simulink model "robotsim"  (Simulink 7.4)
settings: Solver=ode45  StartTime=0.0  StopTime=0.05  FixedStep=0.01  MaxStep=0.01  MinStep=0.001  RelTol=1e-3
values from neighbouring files (symbols this model uses):
  robot = wam    [WAMforcecontrol.m]    (also in batchwamobs.m; controltest.m; feedforward.m; inertia2.m = p560)
  uc = M*y+N    [WAMforcecontrol.m]    (also in controltest.m = y+uest; feedforward.m = M*ddqd(i,:)'+Nd; observerest.m = u(1:n); observerest2.m = u(1:n))
  uest = zeros(n,1)    [WAMforcecontrol.m]    (also in controltest.m = a*out(2*n+1:3*n)+(1-a)*uestold; feedforward.m; outputanal.m = M(:,51:57); paralelcontrol2R.m)
undefined symbols (not defined in the file or in its folder): dummyinput
libraries: roblocks x1
settings Model: Creator=acolome  LastModifiedBy=acolome

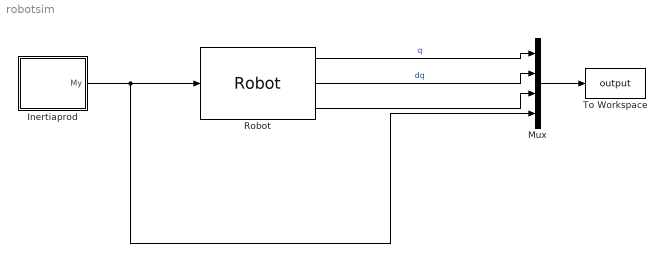
== system robotsim ==
  Inertiaprod : Subsystem  mask{robot=robot, uc=uc, ue=uest}
      mask prompts: robot "Robot Object"
      mask init:
      | n=robot.n
      | trueinput=uc-ue;
      mask Display: port_label('output',1,'u=uc-ue')
  Mux : Mux
  Robot : roblocks/Robot  SystemSampleTime=-1  robot=wam  q0=q0
      link override Integrator1: InitialCondition=q0
  To Workspace : ToWorkspace  VariableName=output  SampleTime=-1  SaveFormat=Array
  wires:
  Mux/1 -> To Workspace/1
  Robot/1 -> Mux/1  "q"
  Robot/2 -> Mux/2  "dq"
  Robot/3 -> Mux/3
  Inertiaprod/1(My) -> Robot/1, Mux/4

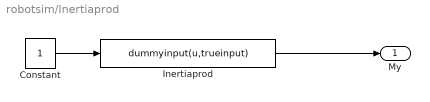
== system robotsim/Inertiaprod ==
  Constant : Constant  OutDataType=fixdt(1, 16)  OutScaling=2^0
  Inertiaprod : MATLABFcn  MATLABFcn=dummyinput(u,trueinput)  OutputDimensions=n
  My : Outport  OutDataType=fixdt(1, 16)  OutScaling=2^0
  wires:
  Inertiaprod/1 -> My/1
  Constant/1 -> Inertiaprod/1
